simulink model "SimpleNeuronTest"  (R2016b)
settings: Solver=ode45  StartTime=0.0  StopTime=5  RelTol=1e-3  EnableMultiTasking=on
libraries: NeuroModelerLibrary x9
settings Model: Creator=Tim  LastModifiedBy=Oleg
settings DataIOCC: LimitDataPoints=on  SaveFormat=Array
settings OptimizationCC: LifeSpan=inf
settings DebuggingCC: SolverPrmCheckMsg=warning  SFUnexpectedBacktrackingDiag=warning  SFNoUnconditionalDefaultTransitionDiag=warning  SFExecutionAtInitializationDiag=none
settings HardwareCC: ProdBitPerPointer=32  ProdBitPerSizeT=32  ProdBitPerPtrDiffT=32  ProdLargestAtomicFloat=None  ProdIntDivRoundTo=Undefined  ProdEndianess=Unspecified  ProdWordSize=32  ProdHWDeviceType=32-bit Generic
settings ModelReferenceCC: PropagateSignalLabelsOutOfModel=off
settings GRTTargetCC: TargetLangStandard=C89/C90 (ANSI)  GeneratePreprocessorConditionals=Disable all
settings ConfigComp: CovMetricSettings=dw  CovHtmlReporting=on  CovSaveCumulativeToWorkspaceVar=on  CovSaveSingleToWorkspaceVar=on  CovExternalEMLEnable=off  CovSFcnEnable=off

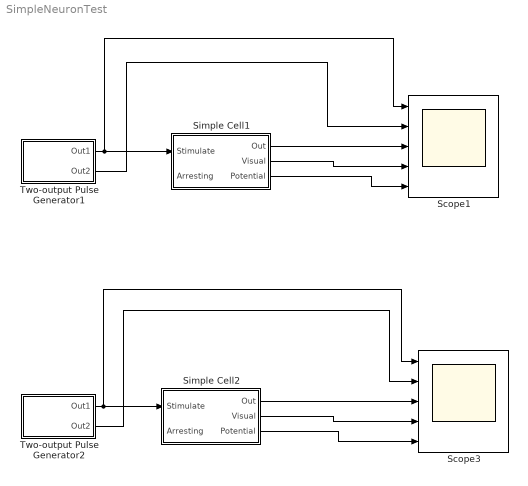
== system SimpleNeuronTest ==
  Scope1 : Scope  NumInputPorts=5
  Scope3 : Scope  NumInputPorts=5
  Simple Cell1 : Subsystem  AncestorBlock=NeuroModelerLibrary/Simple Cells/Simple Cell
  Simple Cell2 : Subsystem  AncestorBlock=NeuroModelerLibrary/Simple Cells/Simple Cell
  Two-output Pulse Generator1 : Subsystem  mask{A=1, P1=400, P2=100, PW=1, ST=0.001, OOn1=0.04, OOff1=3, OOn2=0.4, OOff2=20}
      mask prompts: A "Amplitude"; P1 "Out1: Period (number of samples)"; P2 "Out2: Period (number of samples)"; PW "Pulse Width (number of samples)"; ST "Sample Time"; OOn1 "Out1 On (seconds)"; OOff1 "Out1 Off (seconds)"; OOn2 "Out2 On (seconds)"; OOff2 "Out2 Off (seconds)"
  Two-output Pulse Generator2 : Subsystem  mask{A=1, P1=400, P2=100, PW=1, ST=0.001, OOn1=0.04, OOff1=0.5, OOn2=0.4, OOff2=20}
      mask prompts: A "Amplitude"; P1 "Out1: Period (number of samples)"; P2 "Out2: Period (number of samples)"; PW "Pulse Width (number of samples)"; ST "Sample Time"; OOn1 "Out1 On (seconds)"; OOff1 "Out1 Off (seconds)"; OOn2 "Out2 On (seconds)"; OOff2 "Out2 Off (seconds)"
  wires:
  Two-output Pulse Generator1/1(Out1) -> Scope1/1, Simple Cell1/1(Stimulate)
  Simple Cell1/1(Out) -> Scope1/3
  Simple Cell1/2(Visual) -> Scope1/4
  Simple Cell1/3(Potential) -> Scope1/5
  Two-output Pulse Generator2/1(Out1) -> Scope3/1, Simple Cell2/1(Stimulate)
  Two-output Pulse Generator1/2(Out2) -> Scope1/2
  Two-output Pulse Generator2/2(Out2) -> Scope3/2
  Simple Cell2/1(Out) -> Scope3/3
  Simple Cell2/2(Visual) -> Scope3/4
  Simple Cell2/3(Potential) -> Scope3/5

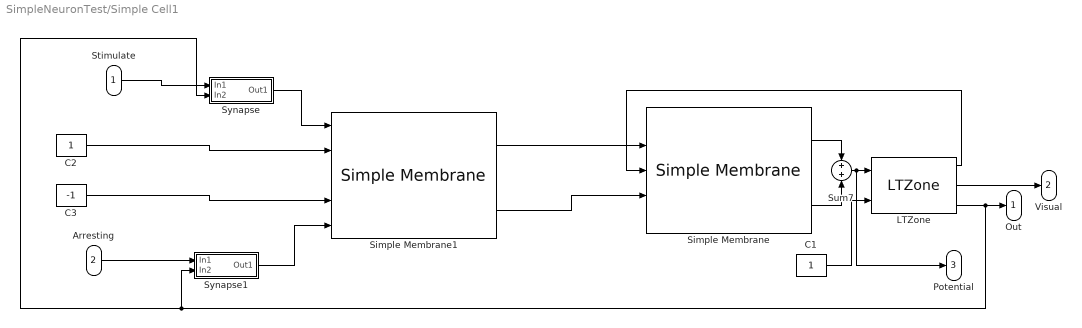
== system SimpleNeuronTest/Simple Cell1 ==
  Stimulate : Inport
  Arresting : Inport  Port=2
  C1 : Constant
  C2 : Constant
  C3 : Constant  Value=-1
  LTZone : NeuroModelerLibrary/Neuron Elements/LTZone  NM=1  FB=1.7  IT=0.005  T=0.001
  Simple Membrane : NeuroModelerLibrary/Neuron Elements/Simple Membrane  ACm=1e-9  ARm=1e7  ECm=1e-9  ERm=1e7  ARFm=1e8  ERFm=1e8
  Simple Membrane1 : NeuroModelerLibrary/Neuron Elements/Simple Membrane  ACm=1e-9  ARm=1e7  ECm=1e-9  ERm=1e7  ARFm=1e8  ERFm=1e8
  Sum7 : Sum  SaturateOnIntegerOverflow=on  InputSameDT=on  OutDataTypeStr=Inherit: Same as first input
  Synapse : Subsystem  AncestorBlock=NeuroModelerLibrary/Neuron Elements/Synapse  mask{SecretionTC=0.001, DecompositionTC=0.01, UseKsi=on, ksi=2, gamma=1e8}
      mask prompts: SecretionTC "Mediator Secretion"; DecompositionTC "Mediator Decomposition"; UseKsi "Use Presynaptic Inhubition"
  Synapse1 : Subsystem  AncestorBlock=NeuroModelerLibrary/Neuron Elements/Synapse  mask{SecretionTC=0.001, DecompositionTC=0.01, UseKsi=on, ksi=2, gamma=1e8}
      mask prompts: SecretionTC "Mediator Secretion"; DecompositionTC "Mediator Decomposition"; UseKsi "Use Presynaptic Inhubition"
  Out : Outport
  Visual : Outport  Port=2
  Potential : Outport  Port=3
  wires:
  LTZone/2 -> Visual/1
  LTZone/3 -> Synapse1/2(In2), Synapse/2(In2), Out/1
  C1/1 -> LTZone/2
  Stimulate/1 -> Synapse/1(In1)
  Arresting/1 -> Synapse1/1(In1)
  Sum7/1 -> LTZone/1, Potential/1
  LTZone/1 -> Simple Membrane/3
  Simple Membrane/1 -> Sum7/1
  Simple Membrane/2 -> Sum7/2
  Simple Membrane1/1 -> Simple Membrane/2
  Simple Membrane1/2 -> Simple Membrane/4
  C3/1 -> Simple Membrane1/4
  C2/1 -> Simple Membrane1/2
  Synapse/1(Out1) -> Simple Membrane1/1
  Synapse1/1(Out1) -> Simple Membrane1/5

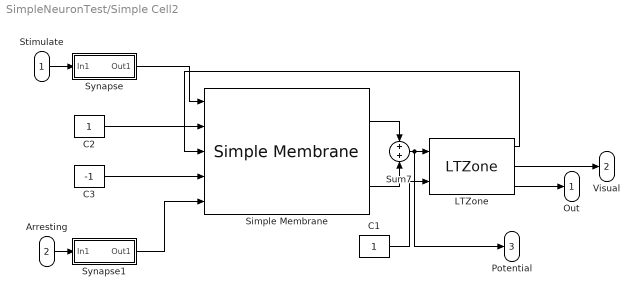
== system SimpleNeuronTest/Simple Cell2 ==
  Stimulate : Inport
  Arresting : Inport  Port=2
  C1 : Constant
  C2 : Constant
  C3 : Constant  Value=-1
  LTZone : NeuroModelerLibrary/Neuron Elements/LTZone  NM=1  FB=1.7  IT=0.005  T=0.001
  Simple Membrane : NeuroModelerLibrary/Neuron Elements/Simple Membrane  ACm=1e-9  ARm=1e7  ECm=1e-9  ERm=1e7  ARFm=1e8  ERFm=1e8
  Sum7 : Sum  SaturateOnIntegerOverflow=on  InputSameDT=on  OutDataTypeStr=Inherit: Same as first input
  Synapse : Subsystem  AncestorBlock=NeuroModelerLibrary/Neuron Elements/Synapse  mask{SecretionTC=0.001, DecompositionTC=0.01, UseKsi=on, ksi=2, gamma=1e8}
      mask prompts: SecretionTC "Mediator Secretion"; DecompositionTC "Mediator Decomposition"; UseKsi "Use Presynaptic Inhubition"
  Synapse1 : Subsystem  AncestorBlock=NeuroModelerLibrary/Neuron Elements/Synapse  mask{SecretionTC=0.001, DecompositionTC=0.01, UseKsi=on, ksi=2, gamma=1e8}
      mask prompts: SecretionTC "Mediator Secretion"; DecompositionTC "Mediator Decomposition"; UseKsi "Use Presynaptic Inhubition"
  Out : Outport
  Visual : Outport  Port=2
  Potential : Outport  Port=3
  wires:
  Synapse1/1(Out1) -> Simple Membrane/5
  Synapse/1(Out1) -> Simple Membrane/1
  Simple Membrane/2 -> Sum7/2
  Simple Membrane/1 -> Sum7/1
  C3/1 -> Simple Membrane/4
  C2/1 -> Simple Membrane/2
  LTZone/1 -> Simple Membrane/3
  Sum7/1 -> Potential/1, LTZone/1
  Arresting/1 -> Synapse1/1(In1)
  Stimulate/1 -> Synapse/1(In1)
  C1/1 -> LTZone/2
  LTZone/3 -> Out/1
  LTZone/2 -> Visual/1

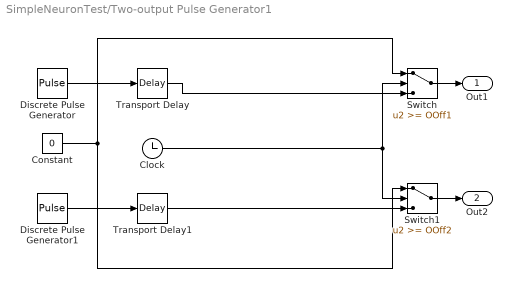
== system SimpleNeuronTest/Two-output Pulse Generator1 ==
  Clock : Clock
  Constant : Constant  Value=0
  Discrete Pulse Generator : DiscretePulseGenerator  Amplitude=A  Period=P1  PulseWidth=PW  SampleTime=ST
  Discrete Pulse Generator1 : DiscretePulseGenerator  Amplitude=A  Period=P2  PulseWidth=PW  SampleTime=ST
  Switch : Switch  Threshold=OOff1  SaturateOnIntegerOverflow=on  InputSameDT=on
  Switch1 : Switch  Threshold=OOff2  SaturateOnIntegerOverflow=on  InputSameDT=on
  Transport Delay : TransportDelay  DelayTime=OOn1
  Transport Delay1 : TransportDelay  DelayTime=OOn2
  Out1 : Outport  InitialOutput=0
  Out2 : Outport  Port=2  InitialOutput=0
  wires:
  Switch1/1 -> Out2/1
  Switch/1 -> Out1/1
  Clock/1 -> Switch1/2, Switch/2
  Transport Delay/1 -> Switch/3
  Transport Delay1/1 -> Switch1/3
  Discrete Pulse Generator1/1 -> Transport Delay1/1
  Constant/1 -> Switch1/1, Switch/1
  Discrete Pulse Generator/1 -> Transport Delay/1

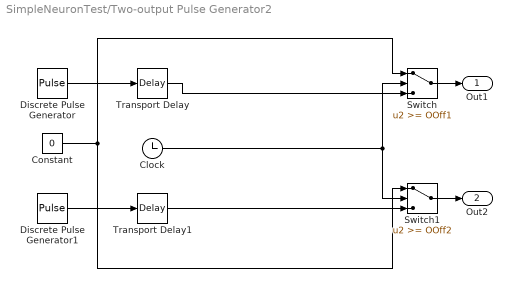
== system SimpleNeuronTest/Two-output Pulse Generator2 ==
  Clock : Clock
  Constant : Constant  Value=0
  Discrete Pulse Generator : DiscretePulseGenerator  Amplitude=A  Period=P1  PulseWidth=PW  SampleTime=ST
  Discrete Pulse Generator1 : DiscretePulseGenerator  Amplitude=A  Period=P2  PulseWidth=PW  SampleTime=ST
  Switch : Switch  Threshold=OOff1  SaturateOnIntegerOverflow=on  InputSameDT=on
  Switch1 : Switch  Threshold=OOff2  SaturateOnIntegerOverflow=on  InputSameDT=on
  Transport Delay : TransportDelay  DelayTime=OOn1
  Transport Delay1 : TransportDelay  DelayTime=OOn2
  Out1 : Outport  InitialOutput=0
  Out2 : Outport  Port=2  InitialOutput=0
  wires:
  Discrete Pulse Generator/1 -> Transport Delay/1
  Constant/1 -> Switch/1, Switch1/1
  Discrete Pulse Generator1/1 -> Transport Delay1/1
  Transport Delay1/1 -> Switch1/3
  Transport Delay/1 -> Switch/3
  Clock/1 -> Switch/2, Switch1/2
  Switch/1 -> Out1/1
  Switch1/1 -> Out2/1

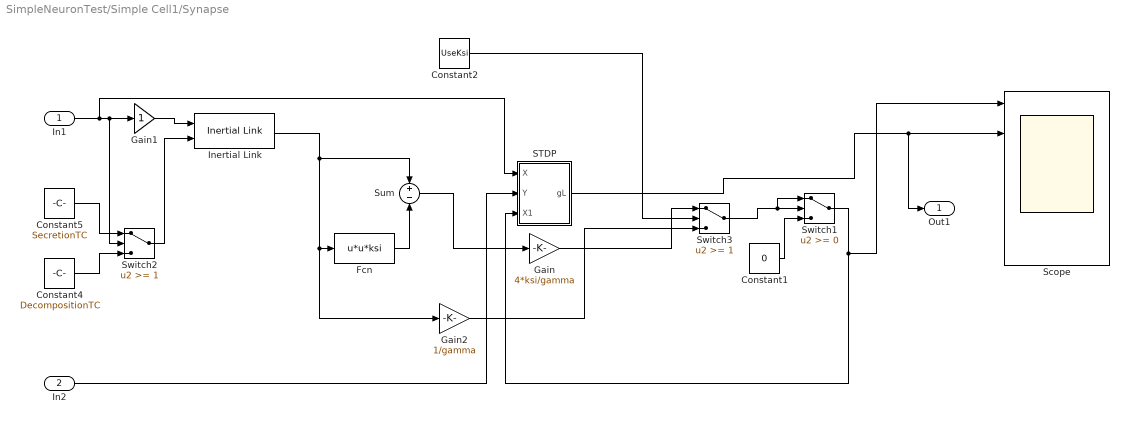
== system SimpleNeuronTest/Simple Cell1/Synapse ==
  In1 : Inport
  In2 : Inport  Port=2
  Constant1 : Constant  Value=0
  Constant2 : Constant  Value=UseKsi
  Constant4 : Constant  Value=DecompositionTC
  Constant5 : Constant  Value=SecretionTC
  Fcn : Fcn  Expr=u*u*ksi
  Gain : Gain  Gain=4*ksi/gamma  SaturateOnIntegerOverflow=on  OutDataTypeStr=Inherit: Same as input  ParamDataTypeStr=Inherit: Same as input
  Gain1 : Gain  SaturateOnIntegerOverflow=on  OutDataTypeStr=Inherit: Same as input  ParamDataTypeStr=Inherit: Same as input
  Gain2 : Gain  Gain=1/gamma  SaturateOnIntegerOverflow=on  OutDataTypeStr=Inherit: Same as input  ParamDataTypeStr=Inherit: Same as input
  Inertial Link : NeuroModelerLibrary/Support/Inertial Link
  STDP : Subsystem
  Scope : Scope  NumInputPorts=6
  Sum : Sum  Inputs=+-  SaturateOnIntegerOverflow=on
  Switch1 : Switch
  Switch2 : Switch  Threshold=1
  Switch3 : Switch  Threshold=1
  Out1 : Outport
  wires:
  Fcn/1 -> Sum/2
  In1/1 -> STDP/1(X), Switch2/2, Gain1/1
  Inertial Link/1 -> Gain2/1, Fcn/1, Sum/1
  Constant4/1 -> Switch2/3
  Constant5/1 -> Switch2/1
  Switch2/1 -> Inertial Link/2
  Constant1/1 -> Switch1/3
  Gain1/1 -> Inertial Link/1
  Switch3/1 -> Switch1/1, Switch1/2
  Constant2/1 -> Switch3/2
  Gain2/1 -> Switch3/3
  In2/1 -> STDP/2(Y)
  Sum/1 -> Gain/1
  Gain/1 -> Switch3/1
  STDP/1(gL) -> Out1/1, Scope/2
  Switch1/1 -> Scope/1, STDP/3(X1)

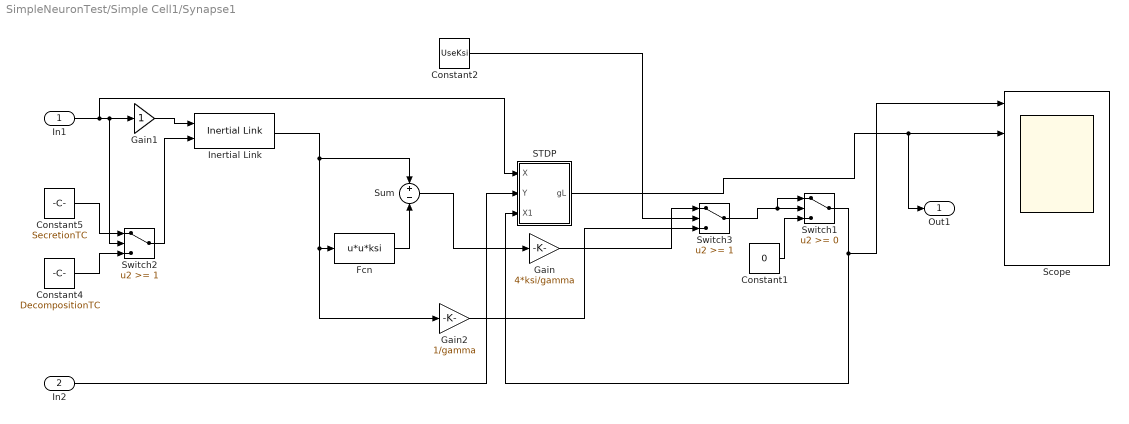
== system SimpleNeuronTest/Simple Cell1/Synapse1 ==
  In1 : Inport
  In2 : Inport  Port=2
  Constant1 : Constant  Value=0
  Constant2 : Constant  Value=UseKsi
  Constant4 : Constant  Value=DecompositionTC
  Constant5 : Constant  Value=SecretionTC
  Fcn : Fcn  Expr=u*u*ksi
  Gain : Gain  Gain=4*ksi/gamma  SaturateOnIntegerOverflow=on  OutDataTypeStr=Inherit: Same as input  ParamDataTypeStr=Inherit: Same as input
  Gain1 : Gain  SaturateOnIntegerOverflow=on  OutDataTypeStr=Inherit: Same as input  ParamDataTypeStr=Inherit: Same as input
  Gain2 : Gain  Gain=1/gamma  SaturateOnIntegerOverflow=on  OutDataTypeStr=Inherit: Same as input  ParamDataTypeStr=Inherit: Same as input
  Inertial Link : NeuroModelerLibrary/Support/Inertial Link
  STDP : Subsystem
  Scope : Scope  NumInputPorts=6
  Sum : Sum  Inputs=+-  SaturateOnIntegerOverflow=on
  Switch1 : Switch
  Switch2 : Switch  Threshold=1
  Switch3 : Switch  Threshold=1
  Out1 : Outport
  wires:
  Fcn/1 -> Sum/2
  In1/1 -> STDP/1(X), Switch2/2, Gain1/1
  Inertial Link/1 -> Gain2/1, Fcn/1, Sum/1
  Constant4/1 -> Switch2/3
  Constant5/1 -> Switch2/1
  Switch2/1 -> Inertial Link/2
  Constant1/1 -> Switch1/3
  Gain1/1 -> Inertial Link/1
  Switch3/1 -> Switch1/1, Switch1/2
  Constant2/1 -> Switch3/2
  Gain2/1 -> Switch3/3
  In2/1 -> STDP/2(Y)
  Sum/1 -> Gain/1
  Gain/1 -> Switch3/1
  STDP/1(gL) -> Out1/1, Scope/2
  Switch1/1 -> Scope/1, STDP/3(X1)

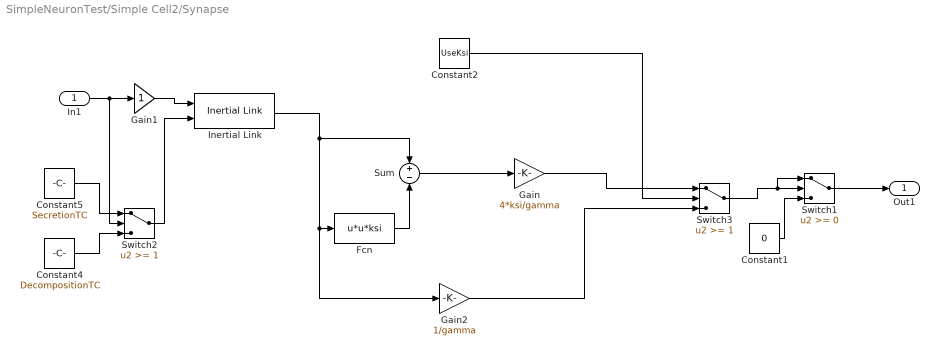
== system SimpleNeuronTest/Simple Cell2/Synapse ==
  In1 : Inport
  Constant1 : Constant  Value=0
  Constant2 : Constant  Value=UseKsi
  Constant4 : Constant  Value=DecompositionTC
  Constant5 : Constant  Value=SecretionTC
  Fcn : Fcn  Expr=u*u*ksi
  Gain : Gain  Gain=4*ksi/gamma  SaturateOnIntegerOverflow=on  OutDataTypeStr=Inherit: Same as input  ParamDataTypeStr=Inherit: Same as input
  Gain1 : Gain  SaturateOnIntegerOverflow=on  OutDataTypeStr=Inherit: Same as input  ParamDataTypeStr=Inherit: Same as input
  Gain2 : Gain  Gain=1/gamma  SaturateOnIntegerOverflow=on  OutDataTypeStr=Inherit: Same as input  ParamDataTypeStr=Inherit: Same as input
  Inertial Link : NeuroModelerLibrary/Support/Inertial Link
  Sum : Sum  Inputs=+-  SaturateOnIntegerOverflow=on
  Switch1 : Switch
  Switch2 : Switch  Threshold=1
  Switch3 : Switch  Threshold=1
  Out1 : Outport
  wires:
  Gain/1 -> Switch3/1
  Gain2/1 -> Switch3/3
  Constant2/1 -> Switch3/2
  Switch3/1 -> Switch1/2, Switch1/1
  Switch1/1 -> Out1/1
  Gain1/1 -> Inertial Link/1
  Constant1/1 -> Switch1/3
  Switch2/1 -> Inertial Link/2
  Constant5/1 -> Switch2/1
  Constant4/1 -> Switch2/3
  Inertial Link/1 -> Sum/1, Fcn/1, Gain2/1
  In1/1 -> Gain1/1, Switch2/2
  Fcn/1 -> Sum/2
  Sum/1 -> Gain/1

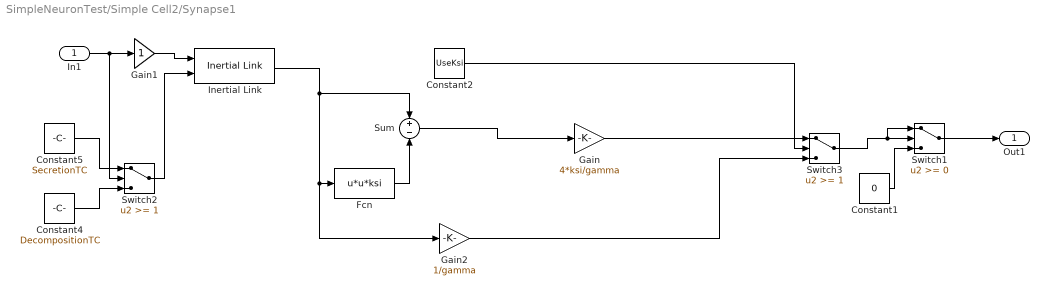
== system SimpleNeuronTest/Simple Cell2/Synapse1 ==
  In1 : Inport
  Constant1 : Constant  Value=0
  Constant2 : Constant  Value=UseKsi
  Constant4 : Constant  Value=DecompositionTC
  Constant5 : Constant  Value=SecretionTC
  Fcn : Fcn  Expr=u*u*ksi
  Gain : Gain  Gain=4*ksi/gamma  SaturateOnIntegerOverflow=on  OutDataTypeStr=Inherit: Same as input  ParamDataTypeStr=Inherit: Same as input
  Gain1 : Gain  SaturateOnIntegerOverflow=on  OutDataTypeStr=Inherit: Same as input  ParamDataTypeStr=Inherit: Same as input
  Gain2 : Gain  Gain=1/gamma  SaturateOnIntegerOverflow=on  OutDataTypeStr=Inherit: Same as input  ParamDataTypeStr=Inherit: Same as input
  Inertial Link : NeuroModelerLibrary/Support/Inertial Link
  Sum : Sum  Inputs=+-  SaturateOnIntegerOverflow=on
  Switch1 : Switch
  Switch2 : Switch  Threshold=1
  Switch3 : Switch  Threshold=1
  Out1 : Outport
  wires:
  Gain2/1 -> Switch3/3
  Constant2/1 -> Switch3/2
  Switch3/1 -> Switch1/2, Switch1/1
  Switch1/1 -> Out1/1
  Gain1/1 -> Inertial Link/1
  Constant1/1 -> Switch1/3
  Switch2/1 -> Inertial Link/2
  Constant5/1 -> Switch2/1
  Constant4/1 -> Switch2/3
  Inertial Link/1 -> Sum/1, Fcn/1, Gain2/1
  In1/1 -> Gain1/1, Switch2/2
  Fcn/1 -> Sum/2
  Gain/1 -> Switch3/1
  Sum/1 -> Gain/1

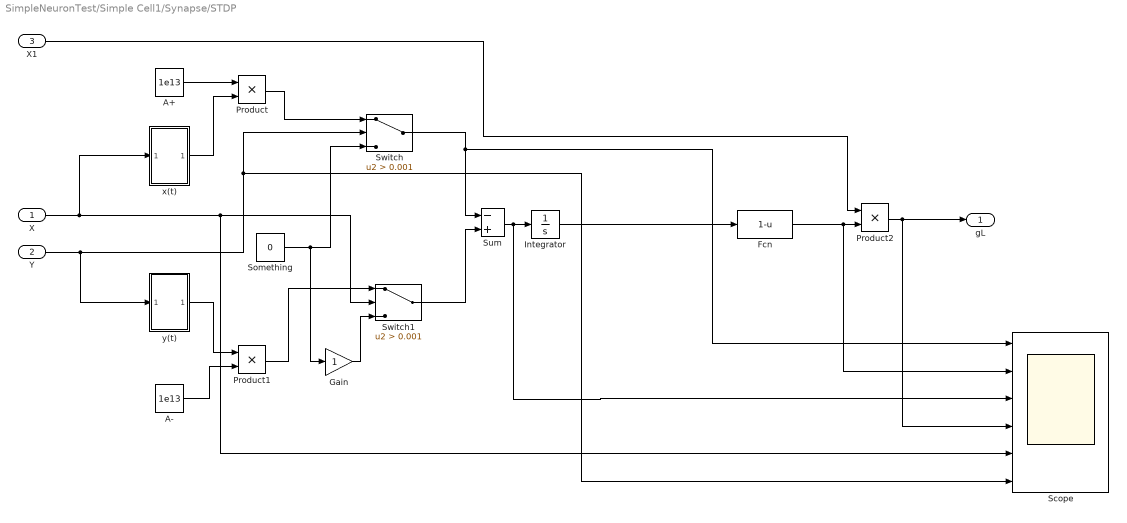
== system SimpleNeuronTest/Simple Cell1/Synapse/STDP ==
  X : Inport
  Y : Inport  Port=2
  X1 : Inport  Port=3
  A+ : Constant  Value=1e13
  A- : Constant  Value=1e13
  Fcn : Fcn  Expr=1-u
  Gain : Gain
  Integrator : Integrator  InitialCondition=1/gamma
  Product : Product
  Product1 : Product
  Product2 : Product
  Scope : Scope  NumInputPorts=6
  Something : Constant  Value=0
  Sum : Sum  Inputs=-+
  Switch : Switch  Criteria=u2 > Threshold  Threshold=0.001
  Switch1 : Switch  Criteria=u2 > Threshold  Threshold=0.001
  "x(t) " : Subsystem
  y(t) : Subsystem
  gL : Outport
  wires:
  Gain/1 -> Switch1/3
  Sum/1 -> Scope/3, Integrator/1
  y(t)/1(Out1) -> Product1/1
  Something/1 -> Switch/3, Gain/1
  Switch/1 -> Sum/1, Scope/1
  "x(t) "/1(Out1) -> Product/2
  Product/1 -> Switch/1
  A+/1 -> Product/1
  Switch1/1 -> Sum/2
  Product1/1 -> Switch1/1
  A-/1 -> Product1/2
  Y/1 -> Switch/2, Scope/6, y(t)/1(In1)
  X/1 -> Scope/5, Switch1/2, "x(t) "/1(In1)
  X1/1 -> Product2/1
  Product2/1 -> Scope/4, gL/1
  Fcn/1 -> Scope/2, Product2/2
  Integrator/1 -> Fcn/1

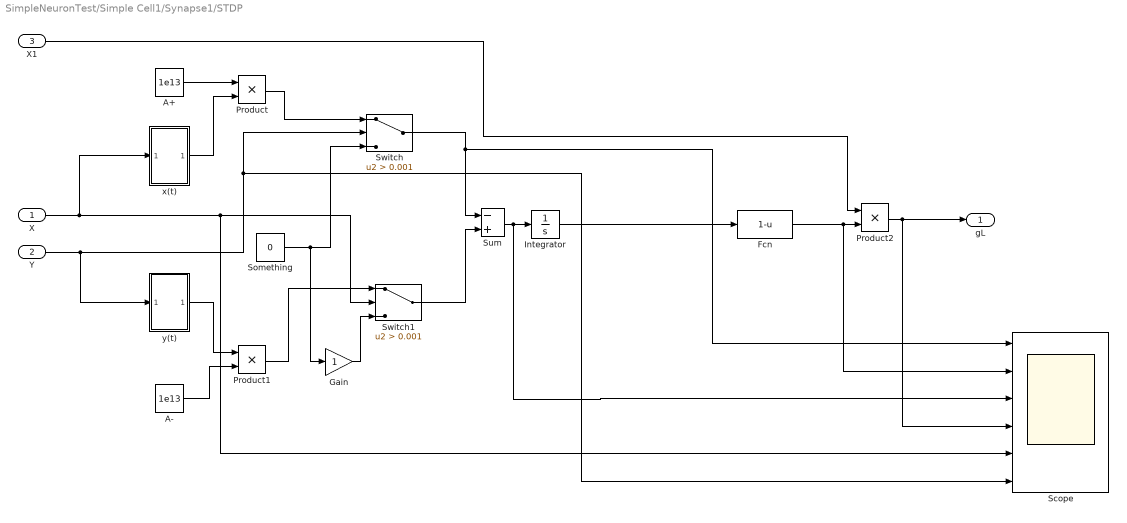
== system SimpleNeuronTest/Simple Cell1/Synapse1/STDP ==
  X : Inport
  Y : Inport  Port=2
  X1 : Inport  Port=3
  A+ : Constant  Value=1e13
  A- : Constant  Value=1e13
  Fcn : Fcn  Expr=1-u
  Gain : Gain
  Integrator : Integrator  InitialCondition=1/gamma
  Product : Product
  Product1 : Product
  Product2 : Product
  Scope : Scope  NumInputPorts=6
  Something : Constant  Value=0
  Sum : Sum  Inputs=-+
  Switch : Switch  Criteria=u2 > Threshold  Threshold=0.001
  Switch1 : Switch  Criteria=u2 > Threshold  Threshold=0.001
  "x(t) " : Subsystem
  y(t) : Subsystem
  gL : Outport
  wires:
  Gain/1 -> Switch1/3
  Sum/1 -> Scope/3, Integrator/1
  y(t)/1(Out1) -> Product1/1
  Something/1 -> Switch/3, Gain/1
  Switch/1 -> Sum/1, Scope/1
  "x(t) "/1(Out1) -> Product/2
  Product/1 -> Switch/1
  A+/1 -> Product/1
  Switch1/1 -> Sum/2
  Product1/1 -> Switch1/1
  A-/1 -> Product1/2
  Y/1 -> Switch/2, Scope/6, y(t)/1(In1)
  X/1 -> Scope/5, Switch1/2, "x(t) "/1(In1)
  X1/1 -> Product2/1
  Product2/1 -> Scope/4, gL/1
  Fcn/1 -> Scope/2, Product2/2
  Integrator/1 -> Fcn/1

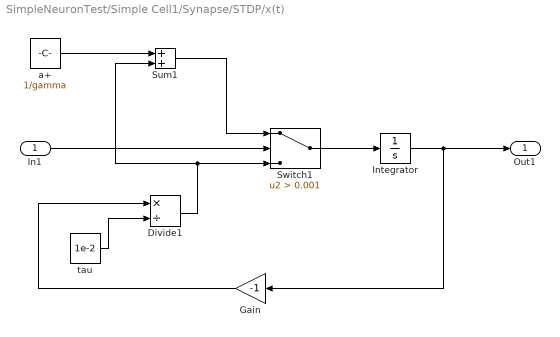
== system SimpleNeuronTest/Simple Cell1/Synapse/STDP/x(t)  ==
  In1 : Inport
  Divide1 : Product  Inputs=*/
  Gain : Gain  Gain=-1
  Integrator : Integrator
  Sum1 : Sum
  Switch1 : Switch  Criteria=u2 > Threshold  Threshold=0.001
  a+ : Constant  Value=1/gamma
  tau : Constant  Value=1e-2
  Out1 : Outport
  wires:
  Switch1/1 -> Integrator/1
  Sum1/1 -> Switch1/1
  Divide1/1 -> Switch1/3, Sum1/2
  tau/1 -> Divide1/2
  Gain/1 -> Divide1/1
  a+/1 -> Sum1/1
  In1/1 -> Switch1/2
  Integrator/1 -> Out1/1, Gain/1

== system SimpleNeuronTest/Simple Cell1/Synapse/STDP/y(t) ==
  In1 : Inport
  Divide1 : Product  Inputs=*/
  Gain : Gain  Gain=-1
  Integrator : Integrator
  Sum1 : Sum
  Switch1 : Switch  Criteria=u2 > Threshold  Threshold=0.001
  a- : Constant  Value=1/gamma
  tau : Constant  Value=1e-3
  Out1 : Outport
  wires:
  Integrator/1 -> Gain/1, Out1/1
  In1/1 -> Switch1/2
  a-/1 -> Sum1/1
  Gain/1 -> Divide1/1
  tau/1 -> Divide1/2
  Divide1/1 -> Sum1/2, Switch1/3
  Sum1/1 -> Switch1/1
  Switch1/1 -> Integrator/1

== system SimpleNeuronTest/Simple Cell1/Synapse1/STDP/x(t)  ==
  In1 : Inport
  Divide1 : Product  Inputs=*/
  Gain : Gain  Gain=-1
  Integrator : Integrator
  Sum1 : Sum
  Switch1 : Switch  Criteria=u2 > Threshold  Threshold=0.001
  a+ : Constant  Value=1/gamma
  tau : Constant  Value=1e-2
  Out1 : Outport
  wires:
  Switch1/1 -> Integrator/1
  Sum1/1 -> Switch1/1
  Divide1/1 -> Switch1/3, Sum1/2
  tau/1 -> Divide1/2
  Gain/1 -> Divide1/1
  a+/1 -> Sum1/1
  In1/1 -> Switch1/2
  Integrator/1 -> Out1/1, Gain/1

== system SimpleNeuronTest/Simple Cell1/Synapse1/STDP/y(t) ==
  In1 : Inport
  Divide1 : Product  Inputs=*/
  Gain : Gain  Gain=-1
  Integrator : Integrator
  Sum1 : Sum
  Switch1 : Switch  Criteria=u2 > Threshold  Threshold=0.001
  a- : Constant  Value=1/gamma
  tau : Constant  Value=1e-3
  Out1 : Outport
  wires:
  Integrator/1 -> Gain/1, Out1/1
  In1/1 -> Switch1/2
  a-/1 -> Sum1/1
  Gain/1 -> Divide1/1
  tau/1 -> Divide1/2
  Divide1/1 -> Sum1/2, Switch1/3
  Sum1/1 -> Switch1/1
  Switch1/1 -> Integrator/1
